simulink model "sdslip1xy"  (Simulink 8.9)
settings: Solver=ode45  StartTime=0.0  StopTime=10  RelTol=1e-5  EnableMultiTasking=on
values from neighbouring files (symbols this model uses):
  k3 = lqrd(a3,b3,eye(3),diag([1 .01/1000]),Ts)    [tslip1.m]
  Kgcar = lqr(Ag1,Bg1,[10 0;0 10],10)    [tslip1.m]
  psii = 0.0    (= 0)    [tslip1.m]
  T0 = 44*(u0/10)^2;Vi(1)=u0    [tslip1.m]
  u0 = x(13)    [smis30.m]    (also in tslip1.m = 5)
  Vi = XU0(1:7)    [tslip1.m]
  xi = 0    [tslip1.m]
  yi = 1    [tslip1.m]
libraries: simulink x1
settings Model: Creator=rodolfo  LastModifiedBy=Pedro
settings DataIOCC: SaveOutput=off  SignalLoggingName=sigsOut
settings OptimizationCC: InitFltsAndDblsToZero=on
settings DebuggingCC: SaveWithParameterizedLinksMsg=none  SignalResolutionControl=TryResolveAllWithWarning  MultiTaskDSMMsg=warning  MultiTaskCondExecSysMsg=none  StateNameClashWarn=none
settings HardwareCC: TargetUnknown=on
settings GRTTargetCC: TargetFcnLib=ansi_tfl_tmw.mat  GeneratePreprocessorConditionals=Use local settings

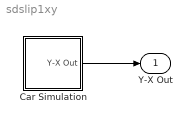
== system sdslip1xy ==
  Car Simulation : Subsystem
  Y-X Out : Outport
  wires:
  Car Simulation/1(Y-X Out) -> Y-X Out/1

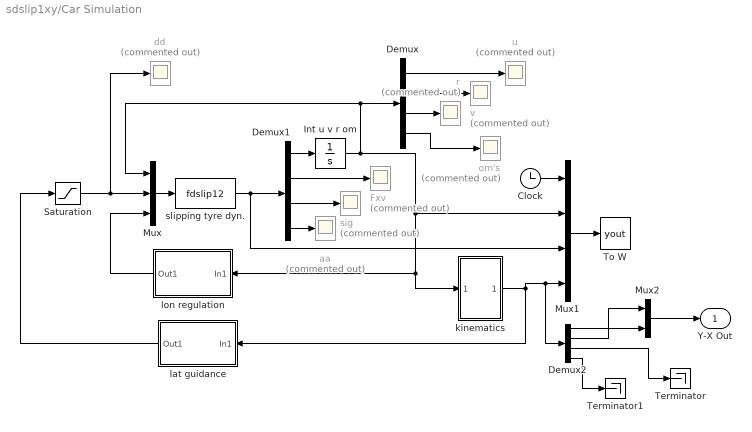
== system sdslip1xy/Car Simulation ==
  Clock : Clock
  Demux : Demux  Outputs=[1 1 1 4]
  Demux1 : Demux  Outputs=[7 4 4 4]
  Demux2 : Demux
  Fxv : Scope  Commented=on
  Int u v r om : Integrator  InitialCondition=Vi
  Mux : Mux  Inputs=[7 1 1]
  Mux1 : Mux  Inputs=[1 7 19 4]
  Mux2 : Mux  Inputs=2
  Saturation : Saturate  UpperLimit=0.69  LowerLimit=-0.69
  Terminator : Terminator
  Terminator1 : Terminator
  To W : ToWorkspace  VariableName=yout  SampleTime=-1
  aa : Scope  Commented=on
  dd : Scope  Commented=on
  kinematics : Subsystem
  lat guidance : Subsystem
  lon regulation : Subsystem
  om's : Scope  Commented=on
  r : Scope  Commented=on
  sig : Scope  Commented=on
  slipping tyre dyn. : MATLABFcn  MATLABFcn=fdslip12  OutputDimensions=3+4+3*4
  u : Scope  Commented=on
  v : Scope  Commented=on
  Y-X Out : Outport
  wires:
  Demux/2 -> v/1
  Demux1/3 -> sig/1
  Demux/4 -> om's/1
  kinematics/1(Out1) -> Demux2/1, Mux1/4, lat guidance/1(In1)
  Demux2/3 -> Terminator/1
  Demux1/2 -> Fxv/1
  Demux/3 -> r/1
  lat guidance/1(Out1) -> Saturation/1
  slipping tyre dyn./1 -> Demux1/1, Mux1/3
  Mux/1 -> slipping tyre dyn./1
  Mux1/1 -> To W/1
  Demux1/1 -> Int u v r om/1
  lon regulation/1(Out1) -> Mux/3
  Demux/1 -> u/1
  Clock/1 -> Mux1/1
  Demux2/4 -> Terminator1/1
  Mux2/1 -> Y-X Out/1
  Demux1/4 -> aa/1
  Int u v r om/1 -> Mux/1, Demux/1, kinematics/1(In1), lon regulation/1(In1), Mux1/2
  Saturation/1 -> dd/1, Mux/2
  Demux2/2 -> Mux2/1
  Demux2/1 -> Mux2/2

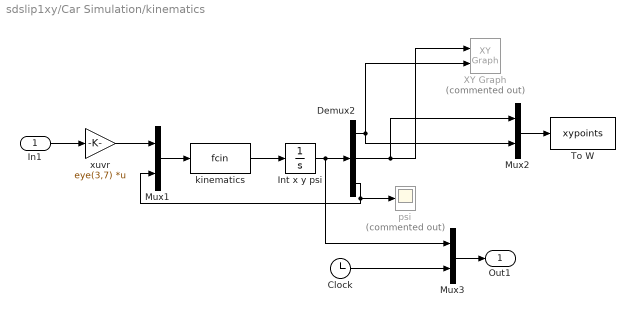
== system sdslip1xy/Car Simulation/kinematics ==
  In1 : Inport
  Clock : Clock
  Demux2 : Demux  Outputs=3
  Int x y psi : Integrator  InitialCondition=[xi yi psii]
  Mux1 : Mux  Inputs=[3 1]
  Mux2 : Mux  Inputs=2
  Mux3 : Mux  Inputs=[3 1]
  To W : ToWorkspace  VariableName=xypoints  SampleTime=-1
  XY Graph : simulink/Sinks/XY Graph  Commented=on  xmin=-30  xmax=30  ymin=-30  ymax=30  st=-1
  kinematics : MATLABFcn  MATLABFcn=fcin  OutputDimensions=3
  psi : Scope  Commented=on
  xuvr : Gain  Gain=eye(3,7)  Multiplication=Matrix(K*u)  SaturateOnIntegerOverflow=on  OutDataTypeStr=Inherit: Same as input  ParamDataTypeStr=Inherit: Same as input
  Out1 : Outport
  wires:
  Mux1/1 -> kinematics/1
  kinematics/1 -> Int x y psi/1
  Int x y psi/1 -> Demux2/1, Mux3/1
  Demux2/3 -> psi/1, Mux1/2
  Demux2/1 -> XY Graph/2, Mux2/2
  Demux2/2 -> XY Graph/1, Mux2/1
  xuvr/1 -> Mux1/1
  In1/1 -> xuvr/1
  Mux2/1 -> To W/1
  Clock/1 -> Mux3/2
  Mux3/1 -> Out1/1

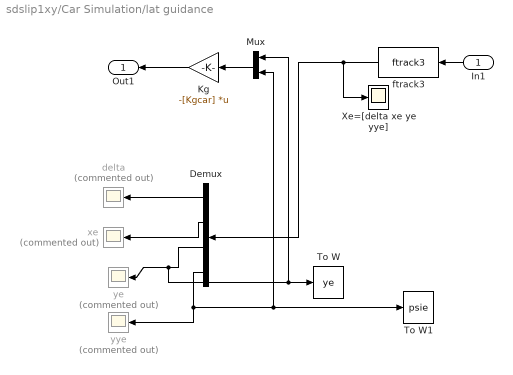
== system sdslip1xy/Car Simulation/lat guidance ==
  In1 : Inport
  Demux : Demux
  Kg : Gain  Gain=-[Kgcar]  Multiplication=Matrix(K*u)  SaturateOnIntegerOverflow=on  OutDataTypeStr=Inherit: Same as input  ParamDataTypeStr=Inherit: Same as input
  Mux : Mux  Inputs=2
  To W : ToWorkspace  VariableName=ye  SampleTime=-1
  To W1 : ToWorkspace  VariableName=psie  SampleTime=-1
  Xe=[delta xe ye yye] : Scope
  delta : Scope  Commented=on
  ftrack3 : MATLABFcn  MATLABFcn=ftrack3  OutputDimensions=4
  xe : Scope  Commented=on
  ye : Scope  Commented=on
  yye : Scope  Commented=on
  Out1 : Outport
  wires:
  ftrack3/1 -> Demux/1, Xe=[delta xe ye yye]/1
  In1/1 -> ftrack3/1
  Demux/2 -> xe/1
  Demux/3 -> ye/1, To W/1, Mux/1
  Demux/1 -> delta/1
  Demux/4 -> yye/1, To W1/1, Mux/2
  Mux/1 -> Kg/1
  Kg/1 -> Out1/1

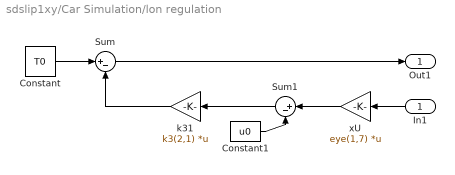
== system sdslip1xy/Car Simulation/lon regulation ==
  In1 : Inport
  Constant : Constant  Value=T0
  Constant1 : Constant  Value=u0
  Sum : Sum  Inputs=|+-  SaturateOnIntegerOverflow=on
  Sum1 : Sum  Inputs=|+-  SaturateOnIntegerOverflow=on
  k31 : Gain  Gain=k3(2,1)  Multiplication=Matrix(K*u)  SaturateOnIntegerOverflow=on  OutDataTypeStr=Inherit: Same as input  ParamDataTypeStr=Inherit: Same as input
  xU : Gain  Gain=eye(1,7)  Multiplication=Matrix(K*u)  SaturateOnIntegerOverflow=on  OutDataTypeStr=Inherit: Same as input  ParamDataTypeStr=Inherit: Same as input
  Out1 : Outport
  wires:
  Constant/1 -> Sum/1
  k31/1 -> Sum/2
  Sum1/1 -> k31/1
  Constant1/1 -> Sum1/2
  xU/1 -> Sum1/1
  In1/1 -> xU/1
  Sum/1 -> Out1/1
